simulink model "Simple_Cruise_control"  (R2012b)
settings: Solver=ode45  StartTime=0.0  StopTime=180  RelTol=1e-3
InitFcn:
  | m=1000;
  | b=50;
  | u=500;
StopFcn:
  | plot(v)
  | grid
libraries: simulink x1
settings Model: Creator=Administrator  LastModifiedBy=Administrator

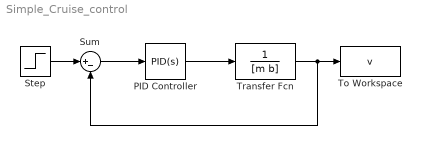
== system Simple_Cruise_control ==
  PID Controller : simulink/Continuous/PID Controller  Controller=PID  TimeDomain=Continuous-time  SampleTime=1  IntegratorMethod=Forward Euler  FilterMethod=Forward Euler  Form=Parallel  P=164.219932905985  I=8.77433253224266  D=-455.885617113905  N=0.360221789723526  InitialConditionSource=internal  InitialConditionForIntegrator=0  InitialConditionForFilter=0  ExternalReset=none  LimitOutput=off  UpperSaturationLimit=inf  LowerSaturationLimit=-inf  LinearizeAsGain=on  AntiWindupMode=none  Kb=1  TrackingMode=off  Kt=1  PParamMin=[]  PParamMax=[]  IParamMin=[]  IParamMax=[]  DParamMin=[]  DParamMax=[]  NParamMin=[]  NParamMax=[]  KbParamMin=[]  KbParamMax=[]  KtParamMin=[]  KtParamMax=[]  POutMin=[]  POutMax=[]  IOutMin=[]  IOutMax=[]  DOutMin=[]  DOutMax=[]  NOutMin=[]  NOutMax=[]  KbOutMin=[]  KbOutMax=[]  KtOutMin=[]  KtOutMax=[]  IntegratorOutMin=[]  IntegratorOutMax=[]  FilterOutMin=[]  FilterOutMax=[]  SumOutMin=[]  SumOutMax=[]  SumI1OutMin=[]  SumI1OutMax=[]  SumI2OutMin=[]  SumI2OutMax=[]  SumI3OutMin=[]  SumI3OutMax=[]  SumDOutMin=[]  SumDOutMax=[]  SaturationOutMin=[]  SaturationOutMax=[]  IntegratorContinuousStateAttributes=''  IntegratorStateMustResolveToSignalObject=off  IntegratorRTWStateStorageClass=Auto  FilterContinuousStateAttributes=''  FilterStateMustResolveToSignalObject=off  FilterRTWStateStorageClass=Auto
  Step : Step  Time=0  Before=10  After=10  SampleTime=0.01
  Sum : Sum  Inputs=|+-
  To Workspace : ToWorkspace  VariableName=v  SampleTime=-1  SaveFormat=Timeseries
  Transfer Fcn : TransferFcn  Denominator=[m b]
  wires:
  Transfer Fcn/1 -> Sum/2, To Workspace/1
  Step/1 -> Sum/1
  PID Controller/1 -> Transfer Fcn/1
  Sum/1 -> PID Controller/1
